simulink model "rotpentemplateV2"  (R2025b)
settings: Solver=ode45  StartTime=0.0  StopTime=run_time  RelTol=1e-3  EnableMultiTasking=on
values from neighbouring files (symbols this model uses):
  adingain = [adingain 1 1 1 1 1]    [hwinit.m]
  adinoffs = [adinoffs 0 0 0 0 0]    [hwinit.m]
  daoutgain = 1*[-6]    [hwinit.m]
  daoutoffs = [0.00]    [hwinit.m]
  h = 0.01    [Multisine_test.m]    (also in animate_pendulum.m = mean(diff(t)); collect_arm2_freeswing.m; collect_freeswing.m; first-script.m)
settings Model: Creator=rbabuska  LastModifiedBy=vincentmaan
settings SolverCC: AlgebraicLoopSolver=TrustRegion
settings DataIOCC: LimitDataPoints=on  SaveFormat=Array  ReturnWorkspaceOutputs=off  SignalLoggingName=sigsOut
settings OptimizationCC: BooleanDataType=off  ExpressionDepthLimit=2147483647.0  InitFltsAndDblsToZero=on  LifeSpan=inf
settings DebuggingCC: SaveWithParameterizedLinksMsg=none  SignalResolutionControl=TryResolveAllWithWarning  MultiTaskDSMMsg=warning  MultiTaskCondExecSysMsg=none  UnconnectedInputMsg=warning  UnconnectedOutputMsg=warning  UnconnectedLineMsg=warning  AllowSymbolicDim=off  StateNameClashWarn=warning  SFUnexpectedBacktrackingDiag=warning  SFNoUnconditionalDefaultTransitionDiag=warning  SFExecutionAtInitializationDiag=none  ArithmeticOperatorsInVariantConditions=warning
settings HardwareCC: ProdBitPerPointer=32.0  ProdBitPerSizeT=32.0  ProdBitPerPtrDiffT=32.0  ProdLargestAtomicFloat=None  ProdIntDivRoundTo=Undefined  ProdEndianess=Unspecified  ProdWordSize=32.0  ProdHWDeviceType=32-bit Generic  TargetUnknown=on
settings ModelReferenceCC: EnableRefExpFcnMdlSchedulingChecks=on  PropagateSignalLabelsOutOfModel=off
settings SFSimCC: SimUseLocalCustomCode=off  CustomCodeUndefinedFunction=UseInterfaceOnly
settings RTWCC: RTWUseLocalCustomCode=off  GPUComputeCapability=3.5  DLArmComputeVersion=19.05
settings CodeAppCC: StateflowObjectComments=on
settings GRTTargetCC: TargetFcnLib=ansi_tfl_tmw.mat  TargetLangStandard=C89/C90 (ANSI)  CombineOutputUpdateFcns=off  GRTInterface=on
settings ConfigComp: CovMetricSettings=dw  CovSaveCumulativeToWorkspaceVar=on  CovSaveSingleToWorkspaceVar=on  CovExternalEMLEnable=off

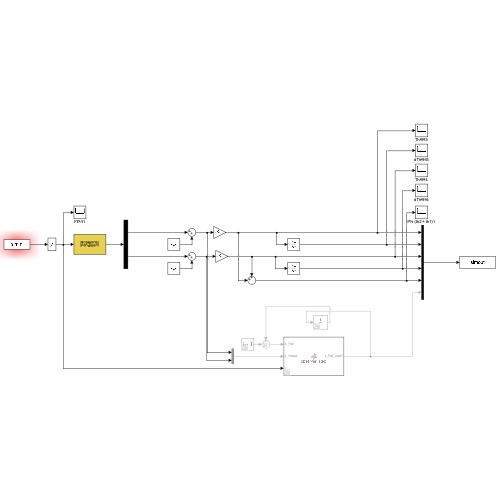
[thumbnail: Simulink's stored preview of the top-level diagram]
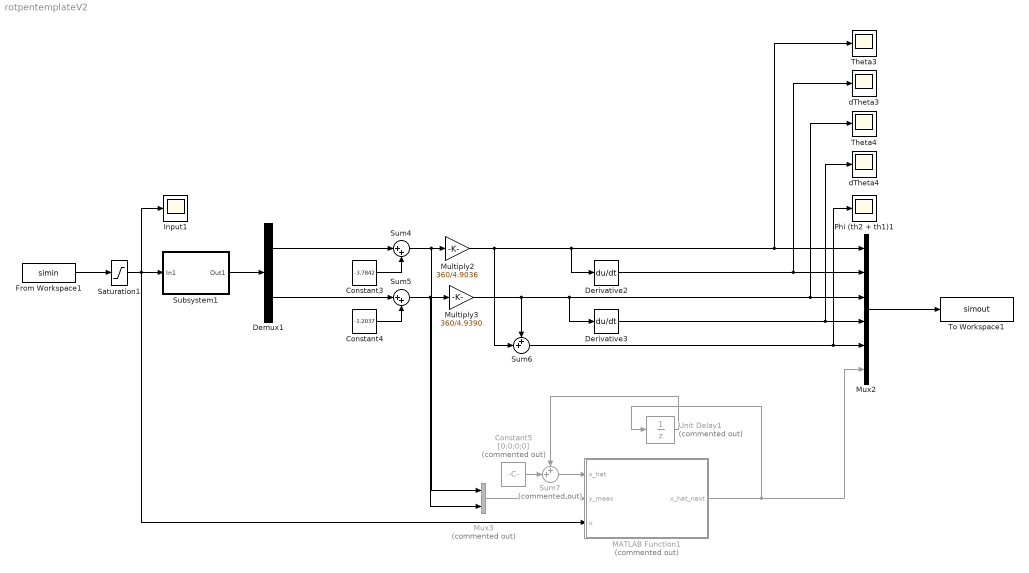
== system rotpentemplateV2 ==
  Constant3 : Constant  Value=-3.7842
  Constant4 : Constant  Value=-1.2037
  Constant5 : Constant  Commented=on  Value=[0;0;0;0]
  Demux1 : Demux  Outputs=2
  Derivative2 : Derivative
  Derivative3 : Derivative
  From Workspace1 : FromWorkspace  VariableName=simin
  Input1 : Scope
      settings: ActiveDisplayYMinimum=-1  ActiveDisplayYMaximum=1  DataLoggingVariableName=ScopeData3
  MATLAB Function1 : MATLAB Function  Commented=on  TreatAsAtomicUnit=on
  Multiply2 : Gain  Gain=360/4.9036
  Multiply3 : Gain  Gain=360/4.9390
  Mux2 : Mux  Inputs=6
  Mux3 : Mux  Commented=on  Inputs=2
  Phi (th2 + th1)1 : Scope
      settings: ActiveDisplayYMinimum=352.5352  ActiveDisplayYMaximum=374.80389  DataLoggingVariableName=ScopeData4
  Saturation1 : Saturate  UpperLimit=1  LowerLimit=-1
  Subsystem1 : Subsystem
      mask Display: disp('Rotational\nPendulum')
  Sum4 : Sum  Inputs=|++
  Sum5 : Sum  Inputs=|++
  Sum6 : Sum  Inputs=++|
  Sum7 : Sum  Commented=on  Inputs=++|
  Theta3 : Scope
      settings: ActiveDisplayYMinimum=-322.81911  ActiveDisplayYMaximum=127.1845  DataLoggingVariableName=ScopeData5
  Theta4 : Scope
      settings: ActiveDisplayYMinimum=-49.9436  ActiveDisplayYMaximum=119.33608  DataLoggingVariableName=ScopeData6
  To Workspace1 : ToWorkspace  VariableName=simout  SaveFormat=Timeseries  SampleTime=-1
  Unit Delay1 : UnitDelay  Commented=on  SampleTime=0.01  HasFrameUpgradeWarning=on
  dTheta3 : Scope
      settings: ActiveDisplayYMinimum=3.78088  ActiveDisplayYMaximum=3.80224  DataLoggingVariableName=ScopeData7
  dTheta4 : Scope
      settings: ActiveDisplayYMinimum=3.78088  ActiveDisplayYMaximum=3.80224  DataLoggingVariableName=ScopeData8
  wires:
  Mux3/1 -> MATLAB Function1/2(y_meas)
  Derivative3/1 -> dTheta4/1, Mux2/4
  Unit Delay1/1 -> Sum7/1
  Sum6/1 -> Phi (th2 + th1)1/1, Mux2/5
  Constant3/1 -> Sum4/2
  Mux2/1 -> To Workspace1/1
  Sum5/1 -> Multiply3/1, Mux3/2
  Sum4/1 -> Mux3/1, Multiply2/1
  Demux1/1 -> Sum4/1
  MATLAB Function1/1(x_hat_next) -> Mux2/6, Unit Delay1/1
  Constant4/1 -> Sum5/2
  Demux1/2 -> Sum5/1
  Sum7/1 -> MATLAB Function1/1(x_hat)
  Saturation1/1 -> Subsystem1/1(In1), Input1/1, MATLAB Function1/3(u)
  Multiply3/1 -> Theta4/1, Mux2/3, Derivative3/1, Sum6/1
  Multiply2/1 -> Theta3/1, Mux2/1, Derivative2/1, Sum6/2
  From Workspace1/1 -> Saturation1/1
  Derivative2/1 -> Mux2/2, dTheta3/1
  Constant5/1 -> Sum7/2
  Subsystem1/1(Out1) -> Demux1/1

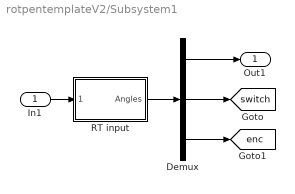
== system rotpentemplateV2/Subsystem1 ==
  In1 : Inport
  Demux : Demux  Outputs=[2 4 1]
  RT input : Subsystem  mask{Ts=h, channels=[6 7]}
      mask prompts: Ts "Sample time [s]:"; channels "Channels to read (e.g., [6 7])"
      mask init:
      | hwinit;
      | 
      | % initialize FPGA
      | fugihandle = fugiboard('Open', 'Pendulum1');
      | fugihandle.WatchdogTimeout = 0.5;
      | fugiboard('SetParams', fugihandle);
      | fugiboard('Write', fugihandle, 0, 0, 0, 0);  % dummy write to sync interface board
      | fugiboard('Write', fugihandle, 5, 1, 0, 0);  % reset position, activate relay
      | data = fugiboard('Read', fugihandle);        % get version info from FPGA
      | % model = bitshift(data(1), -5); 
      | % version = bitand(data(1), 31);
      | % disp(sprintf('FPGA setup %d, version %d', model, version)); % for the B&P it should say 1 1, or else there is a problem
      | fugiboard('Write', fugihandle, 0, 1, 0, 0);  % end reset
      | pause(0.1);                         % give relay some time to respond
      mask Display: disp('Rotational\nPendulum')
  Out1 : Outport
  tag scope: enc=global, switch=global
  wires:
  RT input/1(Angles) -> Demux/1
  Demux/1 -> Out1/1
  Demux/2 -> [switch]
  Demux/3 -> [enc]
  In1/1 -> RT input/1(Motors)

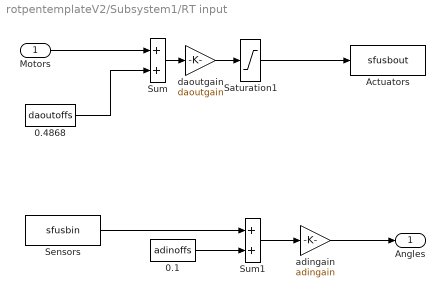
== system rotpentemplateV2/Subsystem1/RT input ==
  Motors : Inport
  0.1 : Constant  Value=adinoffs
  0.4868 : Constant  Value=daoutoffs
  Actuators : S-Function  FunctionName=sfusbout  Parameters=Ts, fugihandle  SFunctionDeploymentMode=off  EnableBusSupport=off
  Saturation1 : Saturate  UpperLimit=10  LowerLimit=-10
  Sensors : S-Function  FunctionName=sfusbin  Parameters=Ts, fugihandle, channels  SFunctionDeploymentMode=off  EnableBusSupport=off
  Sum : Sum  InputSameDT=on  SaturateOnIntegerOverflow=on  OutDataTypeStr=Inherit: Same as first input
  Sum1 : Sum  InputSameDT=on  SaturateOnIntegerOverflow=on  OutDataTypeStr=Inherit: Same as first input
  adingain : Gain  Gain=adingain  SaturateOnIntegerOverflow=on  OutDataTypeStr=Inherit: Same as input  ParamDataTypeStr=Inherit: Same as input
  daoutgain : Gain  Gain=daoutgain  SaturateOnIntegerOverflow=on  OutDataTypeStr=Inherit: Same as input  ParamDataTypeStr=Inherit: Same as input
  Angles : Outport
  wires:
  Sum/1 -> daoutgain/1
  0.4868/1 -> Sum/2
  Motors/1 -> Sum/1
  Sum1/1 -> adingain/1
  0.1/1 -> Sum1/2
  adingain/1 -> Angles/1
  Saturation1/1 -> Actuators/1
  daoutgain/1 -> Saturation1/1
  Sensors/1 -> Sum1/1

== matlab function rotpentemplateV2/MATLAB Function1 ==
  data: x_hat input; y_meas input; u input; x_hat_next output
function x_hat_next = observer_step(x_hat, y_meas, u)


% Inputs:  x_hat  — current state estimate [4x1]
%          y_meas — measured angles [th1; th2]
%          u      — motor input
% Output:  x_hat_next — updated state estimate [4x1]

% These must be defined as persistent or passed as parameters
% Easiest: hardcode them here after computing offline

    h   = 0.01;

    pendulum_params;

    L =  [ 13.2692 2.4922;
         -104.1660 -83.3741;
         -15.9139 0.9017;
          17.9635 165.8050];

    C = [1 0 0 0;
         0 0 1 0];

    % Innovation
    innov = y_meas - C * x_hat;

    % RK4 integration
    k1 = rotpen_ode(0, x_hat,           u, p) + L * (y_meas - C * x_hat);
    k2 = rotpen_ode(0, x_hat+h/2*k1,   u, p) + L * (y_meas - C * (x_hat+h/2*k1));
    k3 = rotpen_ode(0, x_hat+h/2*k2,   u, p) + L * (y_meas - C * (x_hat+h/2*k2));
    k4 = rotpen_ode(0, x_hat+h*k3,     u, p) + L * (y_meas - C * (x_hat+h*k3));

    x_hat_next = x_hat + (h/6)*(k1 + 2*k2 + 2*k3 + k4);

end
